simulink model "prblm4"  (R2020b)
settings: Solver=VariableStepAuto  StartTime=0.0  StopTime=10.0  RelTol=1e-3
undefined symbols (not defined in the file or in its folder): b, J, Kd, Ke, Ki, Kp, Kt, L, R
settings Model: DataDictionary=datadict.sldd  Creator=ANUJA  LastModifiedBy=ANUJA

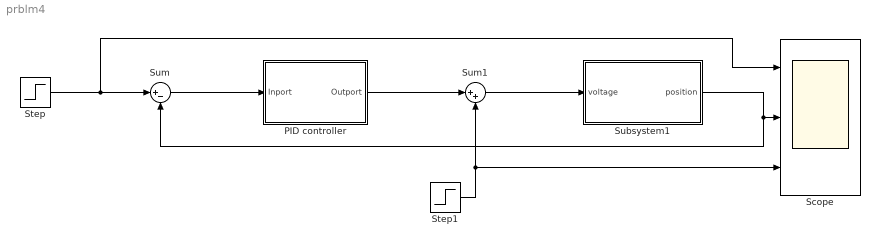
== system prblm4 ==
  PID controller : Subsystem
  Scope : Scope  NumInputPorts=3
  Step : Step  SampleTime=0
  Step1 : Step  SampleTime=0
  Subsystem1 : Subsystem
  Sum : Sum  Inputs=|+-
  Sum1 : Sum  Inputs=|++
  wires:
  Step/1 -> Sum/1, Scope/1
  Sum/1 -> PID controller/1(Inport)
  PID controller/1(Outport) -> Sum1/1
  Sum1/1 -> Subsystem1/1(voltage)
  Subsystem1/1(position) -> Sum/2, Scope/2
  Step1/1 -> Sum1/2, Scope/3

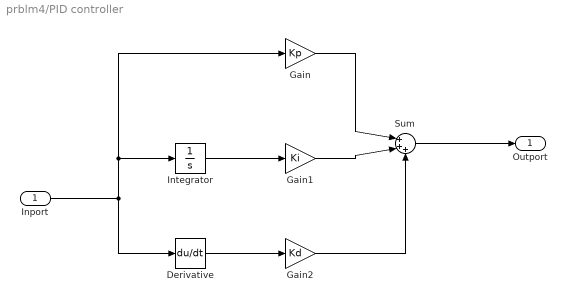
== system prblm4/PID controller ==
  Inport : Inport  OutDataTypeStr=double  PortDimensions=1
  Derivative : Derivative
  Gain : Gain  Gain=Kp
  Gain1 : Gain  Gain=Ki
  Gain2 : Gain  Gain=Kd
  Integrator : Integrator
  Sum : Sum  Inputs=|+++
  Outport : Outport  OutDataTypeStr=double  PortDimensions=1  SampleTime=0
  wires:
  Gain2/1 -> Sum/3
  Sum/1 -> Outport/1
  Derivative/1 -> Gain2/1
  Gain1/1 -> Sum/2
  Inport/1 -> Gain/1, Integrator/1, Derivative/1
  Gain/1 -> Sum/1
  Integrator/1 -> Gain1/1

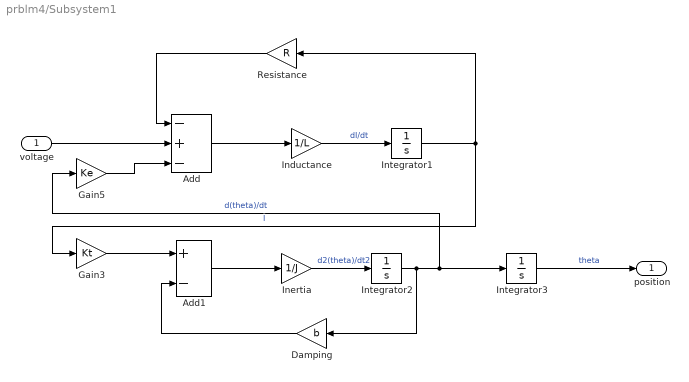
== system prblm4/Subsystem1 ==
  voltage : Inport
  Add : Sum  Inputs=-+-
  Add1 : Sum  Inputs=+-
  Damping : Gain  Gain=b
  Gain3 : Gain  Gain=Kt
  Gain5 : Gain  Gain=Ke
  Inductance : Gain  Gain=1/L
  Inertia : Gain  Gain=1/J
  Integrator1 : Integrator
  Integrator2 : Integrator
  Integrator3 : Integrator
  Resistance : Gain  Gain=R
  position : Outport
  wires:
  voltage/1 -> Add/2
  Integrator2/1 -> Damping/1, Gain5/1, Integrator3/1  "d(theta)/dt"
  Inertia/1 -> Integrator2/1  "d2(theta)/dt2"
  Gain3/1 -> Add1/1
  Add1/1 -> Inertia/1
  Gain5/1 -> Add/3
  Resistance/1 -> Add/1
  Damping/1 -> Add1/2
  Integrator3/1 -> position/1  "theta"
  Integrator1/1 -> Gain3/1, Resistance/1  "I"
  Inductance/1 -> Integrator1/1  "dI/dt"
  Add/1 -> Inductance/1
